simulink model "detection_and_isolation_v2"  (R2018a)
settings: Solver=VariableStepAuto  StartTime=0.0  StopTime=0.8  RelTol=1e-3
values from neighbouring files (symbols this model uses):
  Ad = sysd.A    [SimulinkInit.m]
  Bd = sysd.B    [SimulinkInit.m]
  C1 = Cd(2,:)    [SimulinkInit.m]
  C2 = Cd(3,:)    [SimulinkInit.m]
  C3 = Cd(4,:)    [SimulinkInit.m]
  C4 = Cd(1,:)    [SimulinkInit.m]
  Cd = sysd.C    [SimulinkInit.m]
  T1 = 0.4    [parametros_BIO.m]
  T2 = 1    [parametros_BIO.m]
  T3 = 15    [parametros_BIO.m]
  T4 = 2.5    [parametros_BIO.m]
  tm = 1e-4    (= 0.0001)    [SimulinkInit.m]
undefined symbols (not defined in the file or in its folder): F1, F2, F3, F4, H1, H2, H3, H4, K1U, K2U, K3U, K4U
libraries: powerlib_meascontrol x2, dspstat3 x2
settings Model: Creator=cmparedes  LastModifiedBy=cmparedes

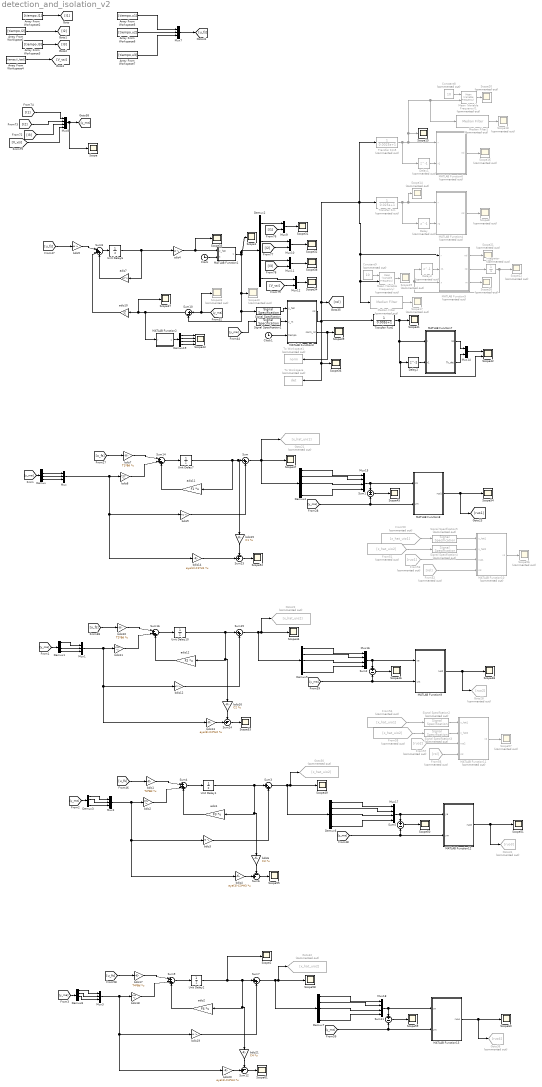
== system detection_and_isolation_v2 ==
  Array From Workspace1 : FromWorkspace  VariableName=[tiempo,I2]  SampleTime=tm
  Array From Workspace2 : FromWorkspace  VariableName=[tiempo,I1]  SampleTime=tm
  Array From Workspace3 : FromWorkspace  VariableName=[tiempo,I3]  SampleTime=tm
  Array From Workspace4 : FromWorkspace  VariableName=[tiempo,V_load]  SampleTime=tm
  Array From Workspace5 : FromWorkspace  VariableName=[tiempo,u1]  SampleTime=tm
  Array From Workspace6 : FromWorkspace  VariableName=[tiempo,u2]  SampleTime=tm
  Array From Workspace7 : FromWorkspace  VariableName=[tiempo,u3]  SampleTime=tm
  Clock : Clock
  Clock1 : Clock
  Constant8 : Constant  Commented=on  Value=10
  Constant9 : Constant  Commented=on  Value=10
  Delay : Delay  Commented=on  DelayLength=1
  Delay1 : Delay  Commented=on  DelayLength=1
  Delay2 : Delay  DelayLength=1
  Delay3 : Delay  Commented=on  DelayLength=1
  Demux{,1..3,8,19} (6 alike) : Demux
  Demux{4..7} (4 alike) : Demux  Outputs=5
  From50 : From  Commented=on  GotoTag=x_hat_uio1
  From51 : From  Commented=on  GotoTag=x_hat_uio2
  From52 : From  Commented=on  GotoTag=rol
  From53 : From  Commented=on  GotoTag=ruo1
  From54 : From  Commented=on  GotoTag=x_hat_uio1
  From55 : From  Commented=on  GotoTag=x_hat_uio2
  From56 : From  Commented=on  GotoTag=rol
  From57 : From  Commented=on  GotoTag=ruo2
  Goto21 : Goto  Commented=on  GotoTag=x_hat_uio1
  Goto22 : Goto  Commented=on  GotoTag=x_hat_uio2
  Goto28 : Goto  Commented=on  GotoTag=ruo2
  Goto30 : Goto  Commented=on  GotoTag=x_hat_uio2
  Goto31 : Goto  Commented=on  GotoTag=ruo3
  Goto32 : Goto  Commented=on  GotoTag=x_hat_uio2
  Goto36 : Goto  Commented=on  GotoTag=ruo4
  Integrator : Integrator  Commented=on
  MATLAB Function1 : MATLAB Function  TreatAsAtomicUnit=on
  MATLAB Function10 : MATLAB Function  Commented=on  TreatAsAtomicUnit=on
  MATLAB Function11 : MATLAB Function  Commented=on  TreatAsAtomicUnit=on
  MATLAB Function12 : MATLAB Function  TreatAsAtomicUnit=on
  MATLAB Function13 : MATLAB Function  TreatAsAtomicUnit=on
  MATLAB Function2 : MATLAB Function  TreatAsAtomicUnit=on
  MATLAB Function3 : MATLAB Function  TreatAsAtomicUnit=on
  MATLAB Function4 : MATLAB Function  Commented=on  TreatAsAtomicUnit=on
  MATLAB Function5 : MATLAB Function  Commented=on  TreatAsAtomicUnit=on
  MATLAB Function6 : MATLAB Function  Commented=on  TreatAsAtomicUnit=on
  MATLAB Function7 : MATLAB Function  TreatAsAtomicUnit=on
  MATLAB Function8 : MATLAB Function  TreatAsAtomicUnit=on
  MATLAB Function9 : MATLAB Function  TreatAsAtomicUnit=on
  Mean (Variable Frequency) : powerlib_meascontrol/Measurements/Mean (Variable Frequency)  Commented=on  Finit=60  Fmin=45  Vinit=0  Ts=0
      settings: SourceProductName=Simscape Power Systems  SourceProductBaseCode=PS
  Mean (Variable Frequency)1 : powerlib_meascontrol/Measurements/Mean (Variable Frequency)  Commented=on  Finit=60  Fmin=45  Vinit=0  Ts=0
      settings: SourceProductName=Simscape Power Systems  SourceProductBaseCode=PS
  Median Filter : dspstat3/Median Filter  Commented=on  WindowLength=100  SimulateUsing=Interpreted execution
      settings: SourceProductName=DSP System Toolbox  SourceProductBaseCode=DS
  Median Filter1 : dspstat3/Median Filter  Commented=on  WindowLength=100  SimulateUsing=Interpreted execution
      settings: SourceProductName=DSP System Toolbox  SourceProductBaseCode=DS
  Mux{,1..3,7} (5 alike) : Mux  Inputs=3
  Mux{9..12,14} (5 alike) : Mux  Inputs=2
  Mux{8,15..18} (5 alike) : Mux
  Scope{,1..2,15,31..32,34..39,41,44..55,58..61} (29 alike) : Scope
  Scope{8,14,16..22,26,33,40,56..57} (14 alike) : Scope  Commented=on
  Scope42 : Scope  NumInputPorts=2
  Scope43 : Scope  NumInputPorts=4
  Signal Specification : SignalSpecification  Dimensions=4
  Signal Specification1 : SignalSpecification  Dimensions=4
  Signal Specification{2..5} (4 alike) : SignalSpecification  Commented=on  Dimensions=3
  Sum{,3,7,15} (4 alike) : Sum  Inputs=|++
  Sum{1..2,5,11} (4 alike) : Sum  Inputs=+-
  Sum10 : Sum  Inputs=|+-
  Sum{6,12,23..24} (4 alike) : Sum  Inputs=-+|
  Sum{4,8..9,14,16} (5 alike) : Sum  Inputs=|+++  SampleTime=tm
  To Workspace : ToWorkspace  Commented=on  VariableName=det  SampleTime=1e-4
  To Workspace1 : ToWorkspace  Commented=on  VariableName=norm  SampleTime=1e-4
  Transfer Fcn : TransferFcn  Commented=on  Denominator=[0.025 1]
  Transfer Fcn5 : TransferFcn  Commented=on  Denominator=[0.0025 1]
  Transfer Fcn6 : TransferFcn  Denominator=[0.005 1]
  Unit Delay{1..2,6..7,10} (5 alike) : UnitDelay  SampleTime=tm
  adis1 : Gain  Gain=F3  Multiplication=Matrix(K*u) (u vector)  SampleTime=tm
  adis10 : Gain  Gain=Ld'  Multiplication=Matrix(K*u) (u vector)  SampleTime=tm
  adis11 : Gain  Gain=F1  Multiplication=Matrix(K*u) (u vector)  SampleTime=tm
  adis12 : Gain  Gain=F2  Multiplication=Matrix(K*u) (u vector)  SampleTime=tm
  adis2 : Gain  Gain=F4  Multiplication=Matrix(K*u) (u vector)  SampleTime=tm
  adis7 : Gain  Gain=Ad  Multiplication=Matrix(K*u) (u vector)  SampleTime=tm
  bdis1 : Gain  Gain=T3*Bd  Multiplication=Matrix(K*u) (u vector)  SampleTime=tm
  bdis10 : Gain  Gain=T2*Bd  Multiplication=Matrix(K*u) (u vector)  SampleTime=tm
  bdis11 : Gain  Gain=K2U  Multiplication=Matrix(K*u) (u vector)  SampleTime=tm
  bdis12 : Gain  Gain=H2  Multiplication=Matrix(K*u) (u vector)  SampleTime=tm
  bdis13 : Gain  Gain=eye(3)-C2*H2  Multiplication=Matrix(K*u) (u vector)  SampleTime=tm
  bdis14 : Gain  Gain=eye(3)-C1*H1  Multiplication=Matrix(K*u) (u vector)  SampleTime=tm
  bdis15 : Gain  Gain=C1  Multiplication=Matrix(K*u) (u vector)  SampleTime=tm
  bdis16 : Gain  Gain=C2  Multiplication=Matrix(K*u) (u vector)  SampleTime=tm
  bdis17 : Gain  Gain=T4*Bd  Multiplication=Matrix(K*u) (u vector)  SampleTime=tm
  bdis18 : Gain  Gain=K4U  Multiplication=Matrix(K*u) (u vector)  SampleTime=tm
  bdis19 : Gain  Gain=H4  Multiplication=Matrix(K*u) (u vector)  SampleTime=tm
  bdis2 : Gain  Gain=K3U  Multiplication=Matrix(K*u) (u vector)  SampleTime=tm
  bdis20 : Gain  Gain=eye(3)-C4*H4  Multiplication=Matrix(K*u) (u vector)  SampleTime=tm
  bdis21 : Gain  Gain=C4  Multiplication=Matrix(K*u) (u vector)  SampleTime=tm
  bdis3 : Gain  Gain=H3  Multiplication=Matrix(K*u) (u vector)  SampleTime=tm
  bdis4 : Gain  Gain=eye(3)-C3*H3  Multiplication=Matrix(K*u) (u vector)  SampleTime=tm
  bdis5 : Gain  Gain=Bd  Multiplication=Matrix(K*u) (u vector)  SampleTime=tm
  bdis6 : Gain  Gain=C3  Multiplication=Matrix(K*u) (u vector)  SampleTime=tm
  bdis7 : Gain  Gain=T1*Bd  Multiplication=Matrix(K*u) (u vector)  SampleTime=tm
  bdis8 : Gain  Gain=K1U  Multiplication=Matrix(K*u) (u vector)  SampleTime=tm
  bdis9 : Gain  Gain=H1  Multiplication=Matrix(K*u) (u vector)  SampleTime=tm
  cdis4 : Gain  Gain=Cd  Multiplication=Matrix(K*u) (u vector)  SampleTime=tm
  wires:
  [V_vsi] -> Mux12/2
  bdis7/1 -> Sum14/1
  Sum5/1 -> Scope50/1
  [V_vsi] -> Mux8/4
  bdis14/1 -> Sum23/2
  Demux7/3 -> Mux18/3
  Array From Workspace3/1 -> [I3]
  adis10/1 -> Sum8/2
  From51/1 -> Signal Specification4/1
  Array From Workspace2/1 -> [I1]
  Demux6/3 -> Mux17/3
  Array From Workspace1/1 -> [I2]
  Sum6/1 -> Scope55/1
  MATLAB Function7/2(Th_det) -> Mux14/2
  Sum23/1 -> Scope52/1
  Demux19/4 -> Scope43/4
  Sum16/1 -> Unit Delay10/1
  bdis15/1 -> Sum23/1
  Signal Specification5/1 -> MATLAB Function10/1(x_hat1)
  MATLAB Function3/1(rol) -> MATLAB Function5/1(r), Median Filter/1, Mean (Variable Frequency)/2, Transfer Fcn5/1, Transfer Fcn/1, [rol], To Workspace/1, Scope36/1, Transfer Fcn6/1
  [u_fs] -> bdis17/1
  MATLAB Function9/1(ruo2) -> Goto28/1, Scope48/1
  MATLAB Function1/1(y) -> Scope1/1, Demux2/1, Scope40/1, Sum10/2, Signal Specification/1
  Signal Specification/1 -> MATLAB Function3/1(y_hat)
  Unit Delay2/1 -> Scope2/1, bdis21/1, adis2/1, Sum7/1
  Demux4/2 -> Mux15/2
  Sum11/1 -> Scope59/1
  From54/1 -> Signal Specification2/1
  Array From Workspace7/1 -> Mux7/3
  Unit Delay10/1 -> bdis16/1, adis12/1, Sum15/1
  MATLAB Function8/1(ruo1) -> [ruo1], Scope54/1
  From53/1 -> MATLAB Function10/3(ruo1)
  Median Filter1/1 -> Scope18/1
  [y_ma] -> Signal Specification1/1
  Demux5/2 -> Mux16/2
  Sum24/1 -> Scope53/1
  adis12/1 -> Sum16/3
  From52/1 -> MATLAB Function10/4(rol)
  Demux2/4 -> Mux12/1
  [I1] -> Mux9/2
  [u_fs] -> bdis1/1
  MATLAB Function5/3(m) -> Scope26/1
  Demux19/3 -> Scope43/3
  [y_ma] -> Sum2/2, MATLAB Function9/2(ym)
  Mux18/1 -> Sum11/1, MATLAB Function13/1(ya)
  Sum8/1 -> Unit Delay6/1
  Demux2/1 -> Mux9/1
  Mean (Variable Frequency)1/1 -> Scope20/1
  Demux5/5 -> Mux16/4
  Mux16/1 -> Sum2/1, MATLAB Function9/1(ya)
  Demux4/5 -> Mux15/4
  Sum15/1 -> Demux5/1, Goto22/1, Scope44/1
  Sum1/1 -> Scope45/1
  Integrator/1 -> Delay3/1, MATLAB Function5/3(x), Scope22/1
  bdis3/1 -> Sum3/2
  Sum10/1 -> MATLAB Function2/1(r), Scope37/1, adis10/1
  Sum12/1 -> Scope61/1
  Delay2/1 -> MATLAB Function7/2(r1)
  bdis1/1 -> Sum4/1
  cdis4/1 -> MATLAB Function1/1(y_hat), Scope35/1
  Array From Workspace6/1 -> Mux7/2
  MATLAB Function2/1(y) -> Demux19/1
  Demux6/2 -> Mux17/2
  Array From Workspace4/1 -> [V_vsi]
  Clock1/1 -> MATLAB Function3/3(tiempo)
  Demux4/3 -> Mux15/3
  [y_ma] -> Sum5/2, MATLAB Function12/2(ym)
  bdis13/1 -> Sum24/2
  Demux6/5 -> Mux17/4
  bdis8/1 -> Sum14/2
  adis7/1 -> Sum8/3
  Mux15/1 -> Sum1/1, MATLAB Function8/1(ya)
  Sum/1 -> Demux4/1, Goto21/1, Scope47/1
  Sum7/1 -> Demux7/1, Goto32/1, Scope58/1
  Demux6/1 -> Mux17/1
  MATLAB Function10/1(v1) -> Scope56/1
  [I3] -> Mux11/2
  Sum3/1 -> Demux6/1, Goto30/1, Scope49/1
  From55/1 -> Signal Specification3/1
  Mux3/1 -> bdis20/1, bdis19/1, bdis18/1
  MATLAB Function12/1(ruo3) -> Goto31/1, Scope51/1
  bdis21/1 -> Sum12/1
  MATLAB Function3/2(norm_rd) -> To Workspace1/1, Scope39/1
  Transfer Fcn5/1 -> Delay1/1, MATLAB Function6/1(r), Median Filter1/1, Mean (Variable Frequency)1/2, Scope15/1
  Mux14/1 -> Scope42/1
  Constant8/1 -> Mean (Variable Frequency)1/1
  From57/1 -> MATLAB Function11/3(ruo2)
  Signal Specification1/1 -> MATLAB Function3/2(y_m)
  Unit Delay1/1 -> bdis6/1, adis1/1, Sum3/1
  MATLAB Function6/1(rol) -> Scope16/1
  Sum9/1 -> Unit Delay2/1
  Unit Delay6/1 -> cdis4/1, adis7/1
  Mux17/1 -> Sum5/1, MATLAB Function12/1(ya)
  Signal Specification2/1 -> MATLAB Function11/1(x_hat1)
  Array From Workspace5/1 -> Mux7/1
  [y_ma] -> Sum11/2, MATLAB Function13/2(ym)
  MATLAB Function11/1(v2) -> Scope57/1
  bdis16/1 -> Sum24/1
  [y_ma] -> Scope33/1, Sum10/1
  Mean (Variable Frequency)/1 -> Scope19/1
  Demux4/1 -> Mux15/1
  Demux2/3 -> Mux11/1
  Mux7/1 -> [u_fs]
  Sum4/1 -> Unit Delay1/1
  Signal Specification3/1 -> MATLAB Function11/2(x_hat2)
  Demux7/5 -> Mux18/4
  Mux1/1 -> bdis13/1, bdis12/1, bdis11/1
  Demux19/2 -> Scope43/2
  bdis9/1 -> Sum/2
  Sum2/1 -> Scope46/1
  Demux7/2 -> Mux18/2
  Unit Delay7/1 -> adis11/1, bdis15/1, Sum/1
  Signal Specification4/1 -> MATLAB Function10/2(x_hat2)
  adis2/1 -> Sum9/3
  Delay1/1 -> MATLAB Function6/2(r1)
  Demux5/3 -> Mux16/3
  adis1/1 -> Sum4/3
  bdis4/1 -> Sum6/2
  Mux9/1 -> Scope31/1
  Median Filter/1 -> Scope17/1
  [I2] -> Mux10/2
  Transfer Fcn/1 -> Delay/1, MATLAB Function4/1(r), Scope14/1
  [I3] -> Mux8/3
  Mux2/1 -> bdis4/1, bdis3/1, bdis2/1
  MATLAB Function7/1(rol) -> Mux14/1
  Delay3/1 -> MATLAB Function5/2(x1)
  Delay/1 -> MATLAB Function4/2(r1)
  Mux12/1 -> Scope34/1
  Demux7/1 -> Mux18/1
  Demux5/1 -> Mux16/1
  bdis20/1 -> Sum12/2
  [u_fs] -> bdis10/1
  Mux8/1 -> Scope/1, [y_ma]
  Constant9/1 -> Mean (Variable Frequency)/1
  bdis12/1 -> Sum15/2
  Sum14/1 -> Unit Delay7/1
  bdis11/1 -> Sum16/2
  [I1] -> Mux8/1
  MATLAB Function5/1(rol) -> Scope21/1
  adis11/1 -> Sum14/3
  bdis18/1 -> Sum9/2
  [u_fs] -> bdis5/1
  Clock/1 -> MATLAB Function1/2(t)
  Mux10/1 -> Scope32/1
  Demux2/2 -> Mux10/1
  MATLAB Function5/2(xp) -> Integrator/1
  Transfer Fcn6/1 -> Scope42/2, Delay2/1, MATLAB Function7/1(r), Scope41/1
  [u_fs] -> bdis7/1
  bdis19/1 -> Sum7/2
  bdis10/1 -> Sum16/1
  MATLAB Function13/1(ruo4) -> Goto36/1, Scope60/1
  Demux19/1 -> Scope43/1
  MATLAB Function4/1(rol) -> Scope8/1
  bdis5/1 -> Sum8/1
  Mux11/1 -> Scope38/1
  bdis6/1 -> Sum6/1
  bdis17/1 -> Sum9/1
  Mux/1 -> bdis14/1, bdis9/1, bdis8/1
  [I2] -> Mux8/2
  [y_ma] -> Sum1/2, MATLAB Function8/2(ym)
  From50/1 -> Signal Specification5/1
  bdis2/1 -> Sum4/2
  From56/1 -> MATLAB Function11/4(rol)
  [y_ma] -> Demux/1
  Demux/2 -> Mux/1
  Demux/3 -> Mux/2
  Demux/4 -> Mux/3
  Demux1/3 -> Mux1/2
  [y_ma] -> Demux1/1
  Demux1/4 -> Mux1/3
  [y_ma] -> Demux3/1
  Demux3/4 -> Mux2/3
  [y_ma] -> Demux8/1
  Demux1/1 -> Mux1/1
  Demux3/1 -> Mux2/1
  Demux3/2 -> Mux2/2
  Demux8/1 -> Mux3/1
  Demux8/2 -> Mux3/2
  Demux8/3 -> Mux3/3

== matlab function detection_and_isolation_v2/MATLAB Function4 ==
  data: r input; rol output; r1 input
function rol = fcn(r,r1)%u1,u2,ym1,ym2)
Th_det = 6.5e-8;
Th_det=0.1;  %2.5

m=r-r1;
if m>0
    Th_det=0.1;  %2.5
elseif m<0 && r<=0.1
    Th_det=0.9; 
end


% sys=tf(1,[0.001 1]);


if r >=Th_det
    rol=1;
else
    rol=0;
end

== matlab function detection_and_isolation_v2/MATLAB Function3 ==
  data: y_hat input; rol output; y_m input; norm_rd output; tiempo input
function [rol,norm_rd] = fcn(y_hat,y_m,tiempo)%u1,u2,ym1,ym2)
Th_det = 6.5e-8;
Th_det=0.07;%2.3e-2; %Funciona bien si los pulsos no estan tan separados
Th_det_up=1;  %2.5 2.25
Th_det_down=-1;
if tiempo >=0.0015 && tiempo <=0.35
    Th_det_up=2.23e-2;  %2.5 2.25
    Th_det_down=3e-4;
else
    Th_det_up=2.25e-2;  %2.5 2.25
    Th_det_down=3e-3;
end
% Th_det=38;
% yol=[u1 ; u2];
% ym=[ym1 ; ym2];

rd1=(y_hat(1)-y_m(1))/100;%200;
rd2=(y_hat(2)-y_m(2))/120;%500;
rd3=(y_hat(3)-y_m(3))/400;%1300; 
rd4=(y_hat(4)-y_m(4))/500;

% rd=y_hat-y_m;
rd=[rd1 rd2 rd3 rd4];
norm_rd=sqrt(sum(rd.^2));
% sys=tf(1,[0.001 1]);


if norm_rd >=Th_det%Th_det_up && norm_rd <=Th_det_down
    rol=1;
else
    rol=0;
end

== matlab function detection_and_isolation_v2/MATLAB Function1 ==
  data: y_hat input; y output; t input
function y = fcn(y_hat,t)%u1,u2,ym1,ym2)
if y_hat(3)>0
    y_hat(3)=y_hat(3)*1.38;
    %     y_hat(3)=y_hat(3)+10;
end

% if t<=0.33
%     y1=y_hat(1)*1;%0.92;
%     y2=y_hat(2)*1;
%     y3=y_hat(3)*1;%1.1; 0.71 0.77 +28
% %     if y3<0
% %         y3=y3+11;
% %     end
%     y4=y_hat(4)*1;%y_hat(4)*1;
%
%
%
% else
%     y1=y_hat(1)*1;%0.92;
%     y2=y_hat(2)*1;
%     y3=y_hat(3)*0.4;%1.1; 0.65; 0.5
%     y4=y_hat(4)*1;%y_hat(4)*1;
% end
if t<=0.33
    y1=y_hat(1)*0.85;
    y2=y_hat(2)*0.8; %0.85
    y3=y_hat(3)*0.57; %0.6
    y4=y_hat(4)*0.88; %0.9
else
    y1=y_hat(1)*0.98;
    y2=y_hat(2)*1.16; %1.13  1.16
    y3=y_hat(3)*0.45; %0.5
    y4=y_hat(4);
    
end

y=[y1 y2 y3 y4];
% if norm_rd >=Th_det
%     rol=1;
% else
%     rol=0;
% end

== matlab function detection_and_isolation_v2/MATLAB Function2 ==
  data: r input; y output
function y = fcn(r)%u1,u2,ym1,ym2)

r1=r(1)/2000;%200;
r2=r(2)/2000;%500;
r3=r(3)/2000;%1300;
r4=r(4)/2000;
y=[r1 r2 r3 r4];
% if norm_rd >=Th_det
%     rol=1;
% else
%     rol=0;
% end

== matlab function detection_and_isolation_v2/MATLAB Function5 ==
  data: r input; rol output; x1 input; xp output; x input; m output
function [rol,xp,m]= fcn(r,x1,x)%u1,u2,ym1,ym2)
Th_det = 6.5e-8;
Th_det=0.1;  %2.5

tao1=0.0025;
tao2=0.0525;
m=x-x1;

% xp= r/tao1-x/tao1;

xp=0;

if m>0
    xp= r/tao1-x/tao1;
    Th_det=0.1;  %2.5
elseif m<0 && x<=0.8
    xp= r/tao2-x/tao2;
    Th_det=0.9; 
end



% sys=tf(1,[0.001 1]);


if x >=Th_det
    rol=1;
else
    rol=0;
end

== matlab function detection_and_isolation_v2/MATLAB Function6 ==
  data: r input; rol output; r1 input
function rol = fcn(r,r1)%u1,u2,ym1,ym2)
Th_det = 6.5e-8;
Th_det=0.1;  %2.5

m=r-r1;
if m>0
    Th_det=0.1;  %2.5
elseif m<0 && r<=0.1
    Th_det=0.9; 
end


% sys=tf(1,[0.001 1]);


if r >=Th_det
    rol=1;
else
    rol=0;
end

== matlab function detection_and_isolation_v2/MATLAB Function7 ==
  data: r input; rol output; r1 input; Th_det output
function [rol,Th_det] = fcn(r,r1)%u1,u2,ym1,ym2)
% Th_det = 6.5e-8;
Th_det=0.08;  %2.5

m=r-r1;
if m>0
    Th_det=0.07;%0.1;  %2.5
elseif m<0 && r<=0.007
    Th_det=0.9; 
end


% sys=tf(1,[0.001 1]);


if r >=Th_det
    rol=1;
else
    rol=0;
end

== matlab function detection_and_isolation_v2/MATLAB Function10 ==
  data: x_hat1 input; v1 output; x_hat2 input; ruo1 input; rol input
function v1 = fcn(x_hat1,x_hat2,ruo1,rol)

% yol=[u1 ; u2];
% ym=[ym1 ; ym2];
 C1=[1     0     0];
 v1=C1*(x_hat1-x_hat2)*ruo1*rol;

== matlab function detection_and_isolation_v2/MATLAB Function11 ==
  data: x_hat1 input; v2 output; x_hat2 input; ruo2 input; rol input
function v2 = fcn(x_hat1,x_hat2,ruo2,rol)

% yol=[u1 ; u2];
% ym=[ym1 ; ym2];
 C2=[0     1     0];
 v2=C2*(x_hat2-x_hat1)*ruo2*rol;

== matlab function detection_and_isolation_v2/MATLAB Function8 ==
  data: ya input; ruo1 output; ym input
function ruo1 = fcn(ya,ym)
Th_uio_on = 3e-3;
Th_uio_off = 1e-5;


Th_uio_on = 6e-3;


% yol=[u1 ; u2];
% ym=[ym1 ; ym2];

% rd1=ya1-ym1;
% rd2=ya2-ym2;

% ya=[ya(1:3)y(5)];
r=ya-ym;

if abs(r(1))  >= Th_uio_on && abs(r(2))  <= Th_uio_off && abs(r(3))  <= Th_uio_off && abs(r(4))  <= Th_uio_off
    ruo1=1;
else
    ruo1=0;
end

== matlab function detection_and_isolation_v2/MATLAB Function9 ==
  data: ya input; ruo2 output; ym input
function ruo2 = fcn(ya,ym)
Th_uio_on = 3e-3;
Th_uio_off = 1e-5;


Th_uio_on = 6e-3;


% yol=[u1 ; u2];
% ym=[ym1 ; ym2];

% rd1=ya1-ym1;
% rd2=ya2-ym2;

% ya=[ya(1:3)y(5)];
r=ya-ym;

if abs(r(1))  >= Th_uio_on && abs(r(2))  <= Th_uio_off && abs(r(3))  <= Th_uio_off && abs(r(4))  <= Th_uio_off
    ruo2=1;
else
    ruo2=0;
end

== matlab function detection_and_isolation_v2/MATLAB Function12 ==
  data: ya input; ruo3 output; ym input
function ruo3 = fcn(ya,ym)
Th_uio_on = 3e-3;
Th_uio_off = 1e-5;


Th_uio_on = 6e-3;


% yol=[u1 ; u2];
% ym=[ym1 ; ym2];

% rd1=ya1-ym1;
% rd2=ya2-ym2;

% ya=[ya(1:3)y(5)];
r=ya-ym;

if abs(r(1))  >= Th_uio_on && abs(r(2))  <= Th_uio_off && abs(r(3))  <= Th_uio_off && abs(r(4))  <= Th_uio_off
    ruo3=1;
else
    ruo3=0;
end

== matlab function detection_and_isolation_v2/MATLAB Function13 ==
  data: ya input; ruo4 output; ym input
function ruo4 = fcn(ya,ym)
Th_uio_on = 3e-3;
Th_uio_off = 1e-5;


Th_uio_on = 6e-3;


% yol=[u1 ; u2];
% ym=[ym1 ; ym2];

% rd1=ya1-ym1;
% rd2=ya2-ym2;

% ya=[ya(1:3)y(5)];
r=ya-ym;

if abs(r(1))  >= Th_uio_on && abs(r(2))  <= Th_uio_off && abs(r(3))  <= Th_uio_off && abs(r(4))  <= Th_uio_off
    ruo4=1;
else
    ruo4=0;
end
